simulink model "LAB_7"  (R2022a)
settings: Solver=VariableStepAuto  StartTime=0.0  StopTime=86400  RelTol=1e-12
libraries: sharedutil x3, matrix_library x1
settings Model: Creator=HAN  LastModifiedBy=이진진
settings DebuggingCC: UnconnectedInputMsg=warning  UnconnectedOutputMsg=warning  UnconnectedLineMsg=warning
settings RTWCC: DLArmComputeVersion=19.05

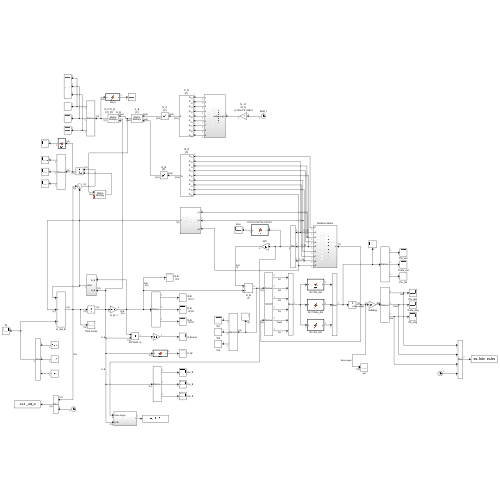
[thumbnail: Simulink's stored preview of the top-level diagram]
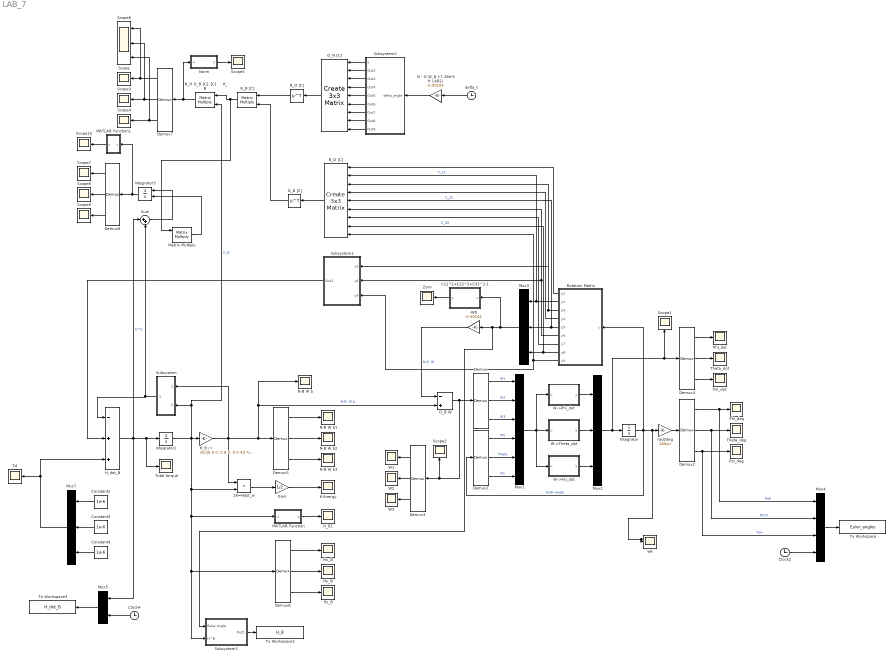
== system LAB_7 ==
  " -W0" : Gain  Gain=-0.00104
  2K=Hdot_w : DotProduct  OutDataTypeStr=Inherit: Inherit via internal rule
  B_O [C] : sharedutil/Create 3x3 Matrix  aMode=aMode
      settings: SourceProductBaseCode=AE,PW,DR,MT,VE
  C12^2+C22^2+C32^2-1 : MATLAB Function  TreatAsAtomicUnit=on
  Clock2 : Clock
  Clock4 : Clock
  Constant2 : Constant  Value=1e-6
  Constant3 : Constant  Value=1e-6
  Constant4 : Constant  Value=1e-6
  Demux{,1..8} (9 alike) : Demux  Outputs=3
      settings: DisplayOption=none
  Gain : Gain  Gain=1/2
  H_B / I : Gain  Gain=inv([6 0 0; 0 8 0; 0 0 4])  Multiplication=Matrix(K*u) (u vector)
  H_B1 : Scope
  H_dot_B : Sum  Inputs=-++
  Hx_B : Scope
  Hy_B : Scope
  Hz_B : Scope
  Integrator : Integrator  InitialCondition=[0 0 0 ]*pi/180
  Integrator1 : Integrator  InitialCondition=[0 0.00104*8 0]
  Integrator3 : Integrator  InitialConditionSource=external
  K-Energy : Scope
  MATLAB Function : MATLAB Function  TreatAsAtomicUnit=on
  MATLAB Function1 : MATLAB Function  TreatAsAtomicUnit=on
  Matrix Multiply : Product  Multiplication=Matrix(*)
  Mux1 : Mux  Inputs=6
  Mux2 : Mux  Inputs=3
  Mux3 : Mux  Inputs=3
  Mux4 : Mux
  Mux5 : Mux  Inputs=2
  Mux7 : Mux  Inputs=3
  N - O W_N (-7.28e-5 fr.LAB1) : Gain  Gain=-0.00104
  N-B W b{,1..3} (4 alike) : Scope
  N_B [C] : Product  Multiplication=Matrix(*)
  N_O [C] : Math  Operator=transpose
  N_O O_B [C]  [C]     H_B : Product  Multiplication=Matrix(*)
  Norm : MATLAB Function  TreatAsAtomicUnit=on
  O_B W : Sum  Inputs=-+
  O_B [C] : Math  Operator=transpose
  O_N [C] : sharedutil/Create 3x3 Matrix  aMode=aMode
      settings: SourceProductBaseCode=AE,PW,DR,MT,VE
  Phi_deg : Scope
  Phi_dot : Scope
  Psi_deg : Scope
  Psi_dot : Scope
  Rotation Matrix : Subsystem
  Scope{,1..5,7..10} (10 alike) : Scope
  Scope6 : Scope  NumInputPorts=3
  Subsystem : Subsystem
  Subsystem1 : Subsystem
  Subsystem2 : Subsystem
  Subsystem3 : Subsystem
  Sum : Sum  Inputs=|++
  Td : Scope
  Theta_deg : Scope
  Theta_dot : Scope
  To Workspace : ToWorkspace  VariableName=Euler_angles  SampleTime=-1
  To Workspace2 : ToWorkspace  VariableName=H_B  SampleTime=-1
  To Workspace3 : ToWorkspace  VariableName=H_dot_B  SampleTime=-1
  Total torque : Scope
  W->Phi_dot : MATLAB Function  TreatAsAtomicUnit=on
  W->Psi_dot : MATLAB Function  TreatAsAtomicUnit=on
  W->Theta_dot : MATLAB Function  TreatAsAtomicUnit=on
  W1 : Scope
  W2 : Scope
  W3 : Scope
  Zero : Scope
  delta_t : Clock
  rad2deg : Gain  Gain=180/pi
  w6 : Scope
  wires:
  " -W0"/1 -> O_B W/1  "N-O  W"
  O_B W/1 -> Scope2/1, Demux3/1, Demux/1
  Demux/1 -> Mux1/1  "W1"
  Demux/2 -> Mux1/2  "W2"
  Demux/3 -> Mux1/3  "W3"
  Demux1/1 -> Mux1/4  "Phi"
  Demux1/2 -> Mux1/5  "Theta"
  Demux1/3 -> Mux1/6  "Psi"
  Mux2/1 -> Scope1/1, Demux4/1, Integrator/1
  rad2deg/1 -> Demux2/1
  Demux3/2 -> W2/1
  Demux3/3 -> W3/1
  Demux3/1 -> W1/1
  Mux1/1 -> W->Psi_dot/1(u), W->Theta_dot/1(u), W->Phi_dot/1(u)
  W->Phi_dot/1(y) -> Mux2/1
  W->Theta_dot/1(y) -> Mux2/2
  W->Psi_dot/1(y) -> Mux2/3
  Rotation Matrix/2(y2) -> B_O [C]/2, Mux3/1  "C_12"
  Rotation Matrix/5(y5) -> B_O [C]/5, Mux3/2  "C_22"
  Rotation Matrix/8(y8) -> B_O [C]/8, Mux3/3  "C_32"
  Mux3/1 -> " -W0"/1, Subsystem3/1(Euler Angle), C12^2+C22^2+C32^2-1/1(u)
  C12^2+C22^2+C32^2-1/1(y) -> Zero/1
  Demux4/1 -> Phi_dot/1
  Demux4/2 -> Theta_dot/1
  Demux4/3 -> Psi_dot/1
  Integrator1/1 -> MATLAB Function/1(u), Subsystem3/2(H^B), Demux6/1, 2K=Hdot_w/2, H_B / I/1, N_O O_B [C]  [C]     H_B/2, Subsystem/2(H_B)  "H_B"
  H_B / I/1 -> 2K=Hdot_w/1, Demux5/1, N-B W b/1, O_B W/2, Subsystem/1(" W_B")  "N-B  W b"
  Demux5/1 -> N-B W b1/1
  Demux5/2 -> N-B W b2/1
  Demux5/3 -> N-B W b3/1
  2K=Hdot_w/1 -> Gain/1
  Gain/1 -> K-Energy/1
  Demux6/1 -> Hx_B/1
  Demux6/2 -> Hy_B/1
  Demux6/3 -> Hz_B/1
  Subsystem/1(WxH) -> H_dot_B/1, Sum/2
  Rotation Matrix/1(y1) -> B_O [C]/1
  Rotation Matrix/3(y3) -> Subsystem1/1(y3), B_O [C]/3
  Rotation Matrix/4(y4) -> B_O [C]/4
  Rotation Matrix/6(y6) -> B_O [C]/6, Subsystem1/2(y6)
  Rotation Matrix/7(y7) -> B_O [C]/7
  Rotation Matrix/9(y9) -> Subsystem1/3(y9), B_O [C]/9
  delta_t/1 -> N - O W_N (-7.28e-5 fr.LAB1)/1
  N - O W_N (-7.28e-5 fr.LAB1)/1 -> Subsystem2/1(delta_angle)
  B_O [C]/1 -> O_B [C]/1
  Subsystem2/1(y) -> O_N [C]/1
  Subsystem2/2(Out2) -> O_N [C]/2
  Subsystem2/3(Out3) -> O_N [C]/3
  Subsystem2/4(Out4) -> O_N [C]/4
  Subsystem2/5(Out5) -> O_N [C]/5
  Subsystem2/6(Out6) -> O_N [C]/6
  Subsystem2/7(Out7) -> O_N [C]/7
  Subsystem2/8(Out8) -> O_N [C]/8
  Subsystem2/9(Out9) -> O_N [C]/9
  O_N [C]/1 -> N_O [C]/1
  N_O [C]/1 -> N_B [C]/1
  O_B [C]/1 -> N_B [C]/2
  Demux7/1 -> Scope/1, Scope6/1
  Demux7/2 -> Scope6/2, Scope3/1
  Demux7/3 -> Scope6/3, Scope4/1
  N_B [C]/1 -> Matrix Multiply/1, N_O O_B [C]  [C]     H_B/1
  N_O O_B [C]  [C]     H_B/1 -> Norm/1(u), Demux7/1
  Norm/1(y) -> Scope5/1
  Matrix Multiply/1 -> Integrator3/2
  Sum/1 -> Integrator3/1
  Integrator3/1 -> MATLAB Function1/1(u), Demux8/1
  Demux8/1 -> Scope7/1
  Demux8/2 -> Scope8/1
  Demux8/3 -> Scope9/1
  MATLAB Function/1(y) -> H_B1/1
  MATLAB Function1/1(y) -> Scope10/1
  Constant3/1 -> Mux7/2
  Constant4/1 -> Mux7/3
  Mux7/1 -> H_dot_B/3, Td/1
  Constant2/1 -> Mux7/1
  Subsystem1/1(Out1) -> H_dot_B/2
  Clock4/1 -> Mux5/2
  H_dot_B/1 -> Mux5/1, Total torque/1, Integrator1/1, Sum/1  "H^b"
  Mux5/1 -> To Workspace3/1
  Subsystem3/1(Out1) -> To Workspace2/1
  Demux2/3 -> Mux4/3, Psi_deg/1  "Yaw"
  Mux4/1 -> To Workspace/1
  Clock2/1 -> Mux4/4
  Demux2/2 -> Mux4/2, Theta_deg/1  "Ptich"
  Demux2/1 -> Mux4/1, Phi_deg/1  "Roll"
  Integrator/1 -> w6/1, rad2deg/1, Rotation Matrix/1(u), Demux1/1  "Euler angle"

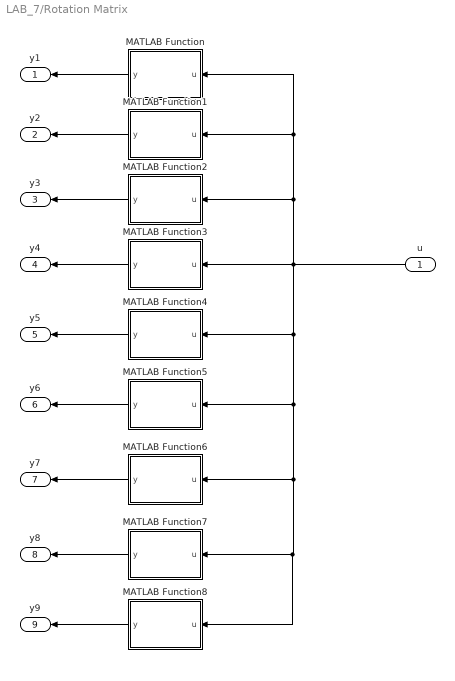
== system LAB_7/Rotation Matrix ==
  u : Inport
  MATLAB Function : MATLAB Function  TreatAsAtomicUnit=on
  MATLAB Function1 : MATLAB Function  TreatAsAtomicUnit=on
  MATLAB Function2 : MATLAB Function  TreatAsAtomicUnit=on
  MATLAB Function3 : MATLAB Function  TreatAsAtomicUnit=on
  MATLAB Function4 : MATLAB Function  TreatAsAtomicUnit=on
  MATLAB Function5 : MATLAB Function  TreatAsAtomicUnit=on
  MATLAB Function6 : MATLAB Function  TreatAsAtomicUnit=on
  MATLAB Function7 : MATLAB Function  TreatAsAtomicUnit=on
  MATLAB Function8 : MATLAB Function  TreatAsAtomicUnit=on
  y1 : Outport
  y2 : Outport  Port=2
  y3 : Outport  Port=3
  y4 : Outport  Port=4
  y5 : Outport  Port=5
  y6 : Outport  Port=6
  y7 : Outport  Port=7
  y8 : Outport  Port=8
  y9 : Outport  Port=9
  wires:
  u/1 -> MATLAB Function8/1(u), MATLAB Function7/1(u), MATLAB Function6/1(u), MATLAB Function5/1(u), MATLAB Function4/1(u), MATLAB Function3/1(u), MATLAB Function1/1(u), MATLAB Function/1(u), MATLAB Function2/1(u)
  MATLAB Function/1(y) -> y1/1
  MATLAB Function1/1(y) -> y2/1
  MATLAB Function2/1(y) -> y3/1
  MATLAB Function3/1(y) -> y4/1
  MATLAB Function4/1(y) -> y5/1
  MATLAB Function5/1(y) -> y6/1
  MATLAB Function6/1(y) -> y7/1
  MATLAB Function7/1(y) -> y8/1
  MATLAB Function8/1(y) -> y9/1

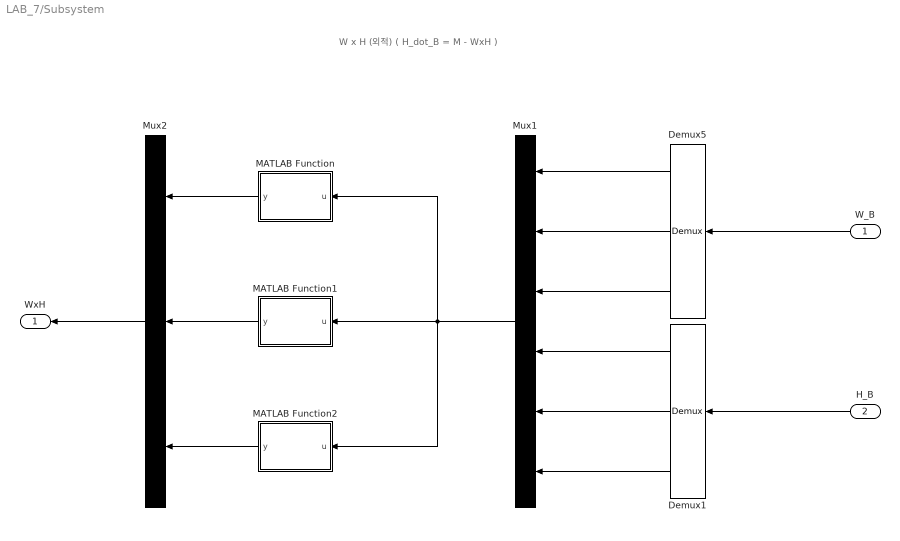
== system LAB_7/Subsystem ==
  note: W x H (외적)
      | ( H_dot_B = M - WxH )
  " W_B" : Inport
  H_B : Inport  Port=2
  Demux1 : Demux  Outputs=3
      settings: DisplayOption=none
  Demux5 : Demux  Outputs=3
      settings: DisplayOption=none
  MATLAB Function : MATLAB Function  TreatAsAtomicUnit=on
  MATLAB Function1 : MATLAB Function  TreatAsAtomicUnit=on
  MATLAB Function2 : MATLAB Function  TreatAsAtomicUnit=on
  Mux1 : Mux  Inputs=6
  Mux2 : Mux  Inputs=3
  WxH : Outport
  wires:
  " W_B"/1 -> Demux5/1
  H_B/1 -> Demux1/1
  Demux5/1 -> Mux1/1
  Demux5/2 -> Mux1/2
  Demux5/3 -> Mux1/3
  Demux1/1 -> Mux1/4
  Demux1/2 -> Mux1/5
  Demux1/3 -> Mux1/6
  Mux1/1 -> MATLAB Function2/1(u), MATLAB Function/1(u), MATLAB Function1/1(u)
  MATLAB Function/1(y) -> Mux2/1
  MATLAB Function1/1(y) -> Mux2/2
  MATLAB Function2/1(y) -> Mux2/3
  Mux2/1 -> WxH/1

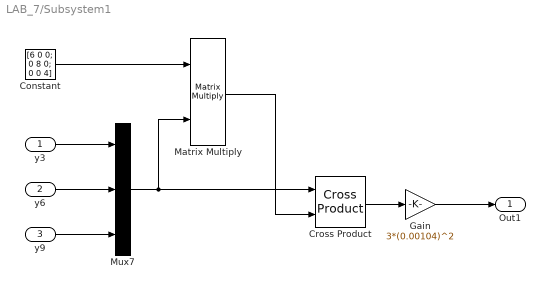
== system LAB_7/Subsystem1 ==
  y3 : Inport
  y6 : Inport  Port=2
  y9 : Inport  Port=3
  Constant : Constant  Value=[6 0 0; 0 8 0; 0 0 4]
  Cross Product : matrix_library/Cross Product
      settings: SourceProductBaseCode=SL
  Gain : Gain  Gain=3*(0.00104)^2
  Matrix Multiply : Product  Multiplication=Matrix(*)
  Mux7 : Mux  Inputs=3
  Out1 : Outport
  wires:
  y3/1 -> Mux7/1
  y6/1 -> Mux7/2
  y9/1 -> Mux7/3
  Constant/1 -> Matrix Multiply/1
  Mux7/1 -> Cross Product/1, Matrix Multiply/2
  Matrix Multiply/1 -> Cross Product/2
  Cross Product/1 -> Gain/1
  Gain/1 -> Out1/1

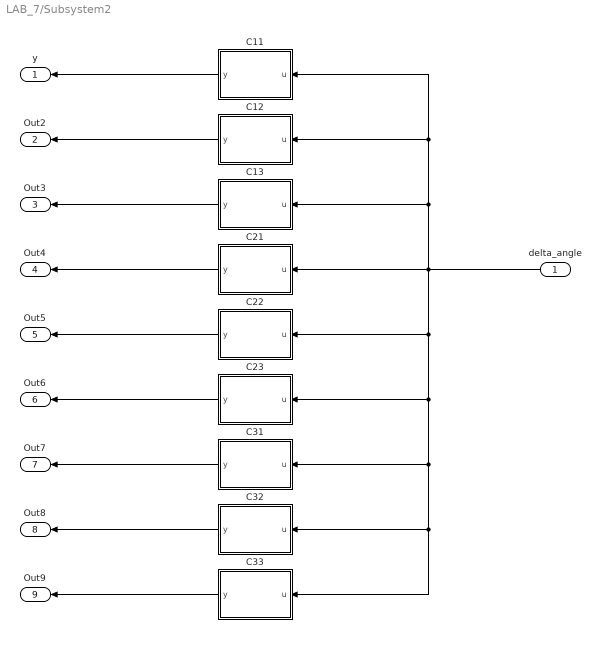
== system LAB_7/Subsystem2 ==
  delta_angle : Inport
  C11 : MATLAB Function  TreatAsAtomicUnit=on
  C12 : MATLAB Function  TreatAsAtomicUnit=on
  C13 : MATLAB Function  TreatAsAtomicUnit=on
  C21 : MATLAB Function  TreatAsAtomicUnit=on
  C22 : MATLAB Function  TreatAsAtomicUnit=on
  C23 : MATLAB Function  TreatAsAtomicUnit=on
  C31 : MATLAB Function  TreatAsAtomicUnit=on
  C32 : MATLAB Function  TreatAsAtomicUnit=on
  C33 : MATLAB Function  TreatAsAtomicUnit=on
  y : Outport
  Out2 : Outport  Port=2
  Out3 : Outport  Port=3
  Out4 : Outport  Port=4
  Out5 : Outport  Port=5
  Out6 : Outport  Port=6
  Out7 : Outport  Port=7
  Out8 : Outport  Port=8
  Out9 : Outport  Port=9
  wires:
  delta_angle/1 -> C33/1(u), C32/1(u), C31/1(u), C23/1(u), C22/1(u), C13/1(u), C12/1(u), C11/1(u), C21/1(u)
  C11/1(y) -> y/1
  C12/1(y) -> Out2/1
  C13/1(y) -> Out3/1
  C21/1(y) -> Out4/1
  C22/1(y) -> Out5/1
  C23/1(y) -> Out6/1
  C31/1(y) -> Out7/1
  C32/1(y) -> Out8/1
  C33/1(y) -> Out9/1

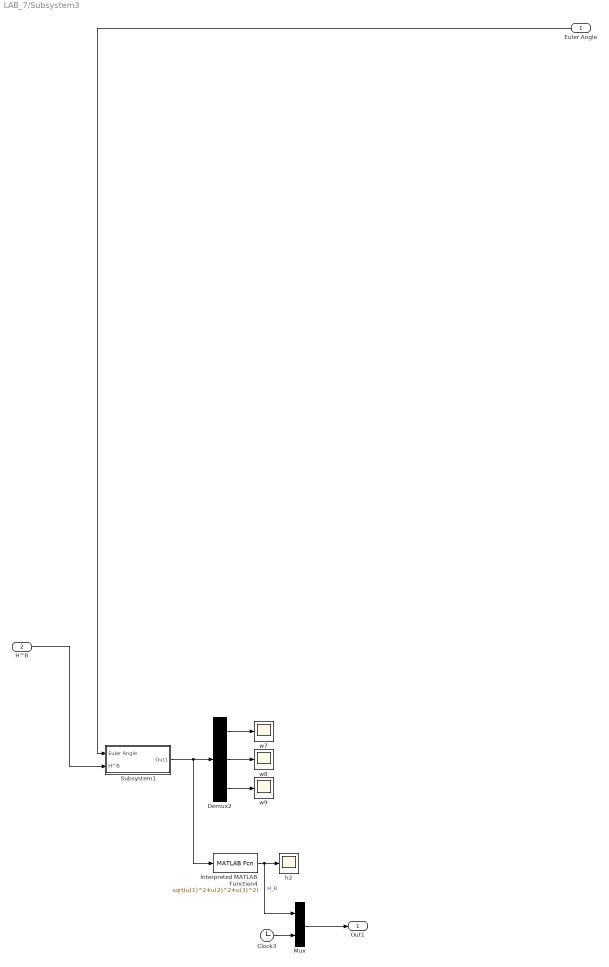
== system LAB_7/Subsystem3 ==
  Euler Angle : Inport
  H^B : Inport  Port=2
  Clock3 : Clock
  Demux2 : Demux  Outputs=3
  Interpreted MATLAB Function4 : MATLABFcn  MATLABFcn=sqrt(u(1)^2+u(2)^2+u(3)^2)
      mask Display: disp('H_B')
  Mux : Mux  Inputs=2
  Subsystem1 : Subsystem
  h2 : Scope
  w7 : Scope
  w8 : Scope
  w9 : Scope
  Out1 : Outport
  wires:
  Interpreted MATLAB Function4/1 -> Mux/1, h2/1  "H_B"
  H^B/1 -> Subsystem1/2(H^B)
  Demux2/1 -> w7/1
  Subsystem1/1(Out1) -> Interpreted MATLAB Function4/1, Demux2/1
  Demux2/3 -> w9/1
  Demux2/2 -> w8/1
  Clock3/1 -> Mux/2
  Euler Angle/1 -> Subsystem1/1(Euler Angle)
  Mux/1 -> Out1/1

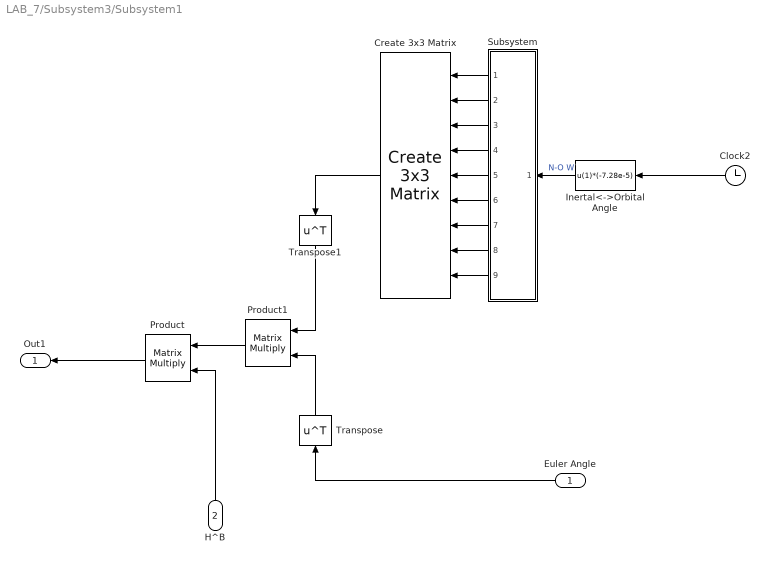
== system LAB_7/Subsystem3/Subsystem1 ==
  Euler Angle : Inport
  H^B : Inport  Port=2
  Clock2 : Clock
  Create 3x3 Matrix : sharedutil/Create 3x3 Matrix  aMode=aMode
      settings: SourceProductBaseCode=AE,PW,DR,MT,VE
  Inertal<->Orbital Angle : Fcn  Expr=u(1)*(-7.28e-5)
  Product : Product  Multiplication=Matrix(*)
  Product1 : Product  Multiplication=Matrix(*)
  Subsystem : Subsystem
  Transpose : Math  Operator=transpose
  Transpose1 : Math  Operator=transpose
  Out1 : Outport
  wires:
  H^B/1 -> Product/2
  Product1/1 -> Product/1
  Inertal<->Orbital Angle/1 -> Subsystem/1(Angle)  "N-O W"
  Subsystem/1(Out1) -> Create 3x3 Matrix/1
  Subsystem/2(Out2) -> Create 3x3 Matrix/2
  Subsystem/4(Out4) -> Create 3x3 Matrix/4
  Subsystem/3(Out3) -> Create 3x3 Matrix/3
  Subsystem/5(Out5) -> Create 3x3 Matrix/5
  Subsystem/6(Out6) -> Create 3x3 Matrix/6
  Subsystem/7(Out7) -> Create 3x3 Matrix/7
  Subsystem/8(Out8) -> Create 3x3 Matrix/8
  Subsystem/9(Out9) -> Create 3x3 Matrix/9
  Create 3x3 Matrix/1 -> Transpose1/1
  Euler Angle/1 -> Transpose/1
  Transpose1/1 -> Product1/1
  Transpose/1 -> Product1/2
  Product/1 -> Out1/1
  Clock2/1 -> Inertal<->Orbital Angle/1

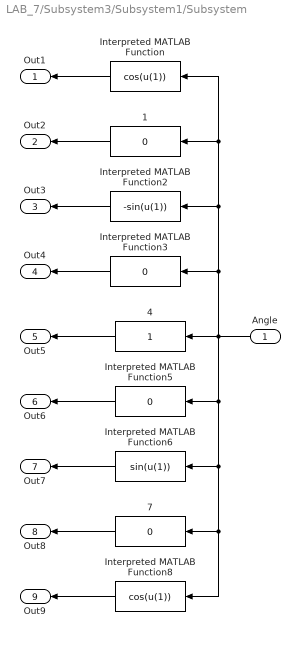
== system LAB_7/Subsystem3/Subsystem1/Subsystem ==
  Angle : Inport
  " 4" : MATLABFcn  MATLABFcn=1
  " 7" : MATLABFcn  MATLABFcn=0
  1 : MATLABFcn  MATLABFcn=0
  Interpreted MATLAB Function : MATLABFcn  MATLABFcn=cos(u(1))
      mask Display: disp('C11')
  Interpreted MATLAB Function2 : MATLABFcn  MATLABFcn=-sin(u(1))
      mask Display: disp('C13')
  Interpreted MATLAB Function3 : MATLABFcn  MATLABFcn=0
      mask Display: disp('C21')
  Interpreted MATLAB Function5 : MATLABFcn  MATLABFcn=0
      mask Display: disp('C23')
  Interpreted MATLAB Function6 : MATLABFcn  MATLABFcn=sin(u(1))
      mask Display: disp('C31')
  Interpreted MATLAB Function8 : MATLABFcn  MATLABFcn=cos(u(1))
      mask Display: disp('C33')
  Out1 : Outport
  Out2 : Outport  Port=2
  Out3 : Outport  Port=3
  Out4 : Outport  Port=4
  Out5 : Outport  Port=5
  Out6 : Outport  Port=6
  Out7 : Outport  Port=7
  Out8 : Outport  Port=8
  Out9 : Outport  Port=9
  wires:
  Interpreted MATLAB Function/1 -> Out1/1
  1/1 -> Out2/1
  Interpreted MATLAB Function2/1 -> Out3/1
  Interpreted MATLAB Function3/1 -> Out4/1
  " 4"/1 -> Out5/1
  Interpreted MATLAB Function5/1 -> Out6/1
  Interpreted MATLAB Function6/1 -> Out7/1
  " 7"/1 -> Out8/1
  Interpreted MATLAB Function8/1 -> Out9/1
  Angle/1 -> " 4"/1, 1/1, Interpreted MATLAB Function/1, Interpreted MATLAB Function2/1, Interpreted MATLAB Function3/1, " 7"/1, Interpreted MATLAB Function8/1, Interpreted MATLAB Function6/1, Interpreted MATLAB Function5/1

== matlab function LAB_7/Subsystem/MATLAB Function1 ==
  data: u input; y output
function y = fcn(u)

y = u(3)*u(4)-u(1)*u(6);

end

== matlab function LAB_7/Subsystem/MATLAB Function2 ==
  data: u input; y output
function y = fcn(u)

y = u(1)*u(5)-u(2)*u(4) ;

end

== matlab function LAB_7/MATLAB Function ==
  data: u input; y output
function y = fcn(u)

y = sqrt(u(1)^2+u(2)^2+u(3)^2);

end

== matlab function LAB_7/Subsystem2/C33 ==
  data: u input; y output
function y = fcn(u)

y = cos(u(1));

end

== matlab function LAB_7/Subsystem2/C32 ==
  data: u input; y output
function y = fcn(u)

y = 0;

end

== matlab function LAB_7/Rotation Matrix/MATLAB Function ==
  data: u input; y output
function y = fcn(u)

y = cos(u(3))*cos(u(2)) ;

end

== matlab function LAB_7/Subsystem2/C31 ==
  data: u input; y output
function y = fcn(u)

y = sin(u(1));

end

== matlab function LAB_7/Subsystem2/C23 ==
  data: u input; y output
function y = fcn(u)

y = 0 ;

end

== matlab function LAB_7/Subsystem2/C22 ==
  data: u input; y output
function y = fcn(u)

y = 1;

end

== matlab function LAB_7/Subsystem2/C21 ==
  data: u input; y output
function y = fcn(u)

y = 0;

end

== matlab function LAB_7/Subsystem2/C13 ==
  data: u input; y output
function y = fcn(u)

y = -sin(u(1));

end

== matlab function LAB_7/Subsystem2/C12 ==
  data: u input; y output
function y = fcn(u)

y = 0;

end

== matlab function LAB_7/Subsystem2/C11 ==
  data: u input; y output
function y = fcn(u)

y = cos(u(1)) ;

end

== matlab function LAB_7/Norm ==
  data: u input; y output
function y = fcn(u)

y = sqrt(u(1)^2+u(2)^2+u(3)^2);

end

== matlab function LAB_7/MATLAB Function1 ==
  data: u input; y output
function y = fcn(u)

y = sqrt(u(1)^2+u(2)^2+u(3)^2);

end

== matlab function LAB_7/Rotation Matrix/MATLAB Function2 ==
  data: u input; y output
function y = fcn(u)

y = -sin(u(2)) ;

end

== matlab function LAB_7/W->Phi_dot ==
  data: u input; y output
function y = fcn(u)

y = u(1) +sin(u(4))*tan(u(5))*u(2) +cos(u(4))*tan(u(5))*u(3) ;

end

== matlab function LAB_7/Rotation Matrix/MATLAB Function3 ==
  data: u input; y output
function y = fcn(u)

y = -sin(u(3))*cos(u(1)) +cos(u(3))*sin(u(2))*sin(u(1)) ;

end

== matlab function LAB_7/Rotation Matrix/MATLAB Function4 ==
  data: u input; y output
function y = fcn(u)

y = cos(u(3))*cos(u(1)) +sin(u(3))*sin(u(2))*sin(u(1)) ; 

end

== matlab function LAB_7/Rotation Matrix/MATLAB Function5 ==
  data: u input; y output
function y = fcn(u)

y = cos(u(2))*sin(u(1)) ;

end

== matlab function LAB_7/Rotation Matrix/MATLAB Function6 ==
  data: u input; y output
function y = fcn(u)

y = sin(u(3))*sin(u(1)) +cos(u(3))*sin(u(2))*cos(u(1)) ;

end

== matlab function LAB_7/Rotation Matrix/MATLAB Function7 ==
  data: u input; y output
function y = fcn(u)

y = -cos(u(3))*sin(u(1)) +sin(u(3))*sin(u(2))*cos(u(1)) ;

end

== matlab function LAB_7/Rotation Matrix/MATLAB Function1 ==
  data: u input; y output
function y = fcn(u)

y = sin(u(3))*cos(u(2)) ;

end

== matlab function LAB_7/Rotation Matrix/MATLAB Function8 ==
  data: u input; y output
function y = fcn(u)

y = cos(u(2))*cos(u(1)) ;

end

== matlab function LAB_7/W->Theta_dot ==
  data: u input; y output
function y = fcn(u)

y = cos(u(4))*u(2) -sin(u(4))*u(3) ;

end

== matlab function LAB_7/W->Psi_dot ==
  data: u input; y output
function y = fcn(u)

y = sin(u(4))/cos(u(5))*u(2) + cos(u(4))/cos(u(5))*u(3) ;

end

== matlab function LAB_7/C12^2+C22^2+C32^2-1 ==
  data: u input; y output
function y = fcn(u)

y = u(1)^2+u(2)^2+u(3)^2 -1 ;

end

== matlab function LAB_7/Subsystem/MATLAB Function ==
  data: u input; y output
function y = fcn(u)

y = u(2)*u(6)-u(3)*u(5) ;

end
